simulink model "PlantaFuzzy1"  (R2023a)
settings: Solver=VariableStepAuto  StartTime=0.0  StopTime=inf  RelTol=1e-3
libraries: fuzblock x1
settings Model: Creator=DELL  LastModifiedBy=DELL

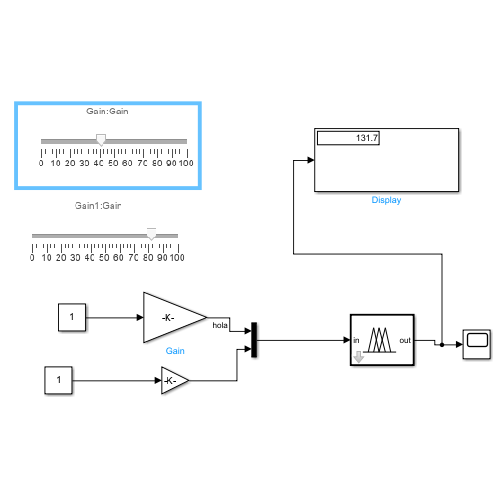
[thumbnail: Simulink's stored preview of the top-level diagram]
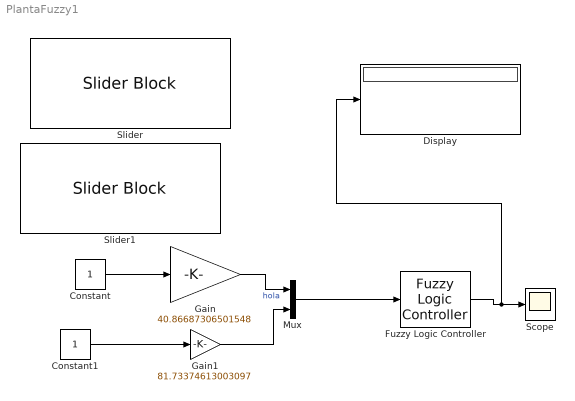
== system PlantaFuzzy1 ==
  Constant : Constant
  Constant1 : Constant
  Display : Display
  Fuzzy Logic Controller : fuzblock/Fuzzy Logic  Controller  FIS='PlantaFuzzy.fis'  OutputSampleNumber=101  DataType=double  FuzzifiedInputs=off  RuleFiringStrengths=off  RuleOutputs=off  AggregatedOutputs=off  SimulateUsing=Interpreted execution  OutOfRangeInputValueMessage=warning  NoRuleFiredMessage=warning  EmptyOutputFuzzySetMessage=warning
  Gain : Gain  Gain=40.86687306501548
  Gain1 : Gain  Gain=81.73374613003097
  Mux : Mux  Inputs=2
  Scope : Scope
  Slider : SliderBlock
  Slider1 : SliderBlock
  wires:
  Mux/1 -> Fuzzy Logic Controller/1
  Fuzzy Logic Controller/1 -> Display/1, Scope/1
  Constant/1 -> Gain/1
  Gain/1 -> Mux/1  "hola"
  Constant1/1 -> Gain1/1
  Gain1/1 -> Mux/2
